simulink model "cic_filter_test9"  (Simulink 7.4)
settings: Solver=ode45  StartTime=0.0  StopTime=1000  RelTol=1e-3
libraries: xbsIndex_r4 x182, xrbsComm_r4 x1, xps_library x1, simulink x1
(part 1 of 2)
settings Model: Creator=chenhong  LastModifiedBy=chenhong

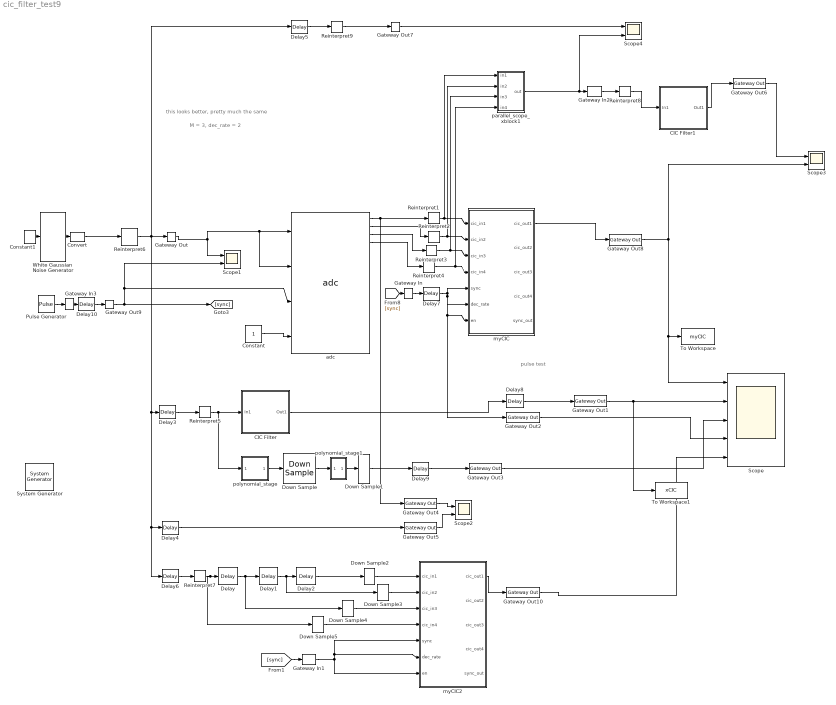
== system cic_filter_test9 ==
  note: pulse test
  note: this looks better, pretty much the same
  note: M = 3, dec_rate = 2
  " System Generator" : xbsIndex_r4/ System Generator  Tag=genX  SystemSampleTime=-1  xilinxfamily=Virtex6  part=xc6vsx315t  speed=-3  package=ff1156  synthesis_tool=XST  clock_wrapper=Clock Enables  directory=./netlist  testbench=off  simulink_period=1  sysclk_period=10  dcm_input_clock_period=10  incr_netlist=off  trim_vbits=Everywhere in SubSystem  dbl_ovrd=According to Block Masks  core_generation=According to Block Masks  run_coregen=off  deprecated_control=off  eval_field=0  block_type=sysgen
      settings: block_version=11.4
  CIC Filter : Subsystem  mask(CIC Filter){input_bitwidth=8, input_binpt=3, filter_type=Decimator, rate_change=4, stages=3, m=1, pipeline=on}
      mask prompts: input_bitwidth "Input Bit Width"; input_binpt "Input Binary Point"; filter_type "Filter Type"; rate_change "Sample Rate Change"; stages "Number of Stages"; m "Differential Delay"; pipeline "Pipeline Differentiators"
      mask help: Cascaded Integrated Comb (CIC) Filter
      mask init:
      | % CIC Single Channel v1.0
      | % Set Block Logo
      | sav_gcb=gcb;
      | [bg,fg] = xlcmap('XBlock',0);
      | iPos = get_param(sav_gcb,'Position');
      | iWidth=iPos(3)-iPos(1); iHeight=iPos(4)-iPos(2);
      | iCx=iWidth/2;
      | iCy=iHeight/2;
      | [logoX, logoY] = xlogo(iPos);
      | 
      | % Determine previous filter type and number of stages
      | prev_stages_list = find_system(sav_gcb, 'lookUnderMasks', 'all', 'FollowLinks', 'on', 'Regexp', 'on', 'Name', '^Integrator*'); %this is a cell array
      | prev_stages = length(prev_stages_list);
      | 
      | prev_filter_list = find_system(sav_gcb, 'lookUnderMasks', 'all', 'FollowLinks', 'on', 'Regexp', 'on', 'Name', '^Up Sample*'); %this is a cell array
      | if (isempty(prev_filter_list))
      |     prev_filter_list = find_system(sav_gcb, 'lookUnderMasks', 'all', 'FollowLinks', 'on', 'Regexp', 'on', 'Name', '^Down Sample*'); %this is a cell array
      |     if (isempty(prev_filter_list))
      |         errordlg('Previous Filter Type could not be determined')
      |     else
      |         prev_filter_type = 2;
      |     end
      | else
      |     prev_filter_type = 1;
      | end
      |   
      |   
      | % Print label on the block
      | if(filter_type == 2)
      |    cic_str = sprintf('%d-Stage\n CIC\n%d:1 Decimator',stages, rate_change);
      | else
      |    cic_str = sprintf('%d-Stage\n CIC\n1:%d Interpolator',stages, rate_change);	
      | end
      | 
      | % Make sure the entered values for stages and channels are positive integers
      | nstages = round(sum(abs(stages)));
      | 
      | % issue an error if the number of stages entered is zero
      | if (nstages == 0)
      | 	nstages = prev_stages;
      | 	errordlg('Number of Stages must be more than zero')
      | end
      | 
      | if (nstages == prev_stages) & (filter_type == prev_filter_type)
      |     return
      | end
      | 
      | if(filter_type == 2) % Decimator
      |    if (prev_filter_type == 1) % was interpolator so turn to decimator
      |        for i= 2:prev_stages,
      | 	      delete_line(sav_gcb, ['Integrator' int2str(i-1) '/' int2str(1)], ['Integrator' int2str(i) '/' int2str(1)]);
      | 	      delete_line(sav_gcb, ['Differentiator' int2str(i-1) '/' int2str(1)], ['Differentiator' int2str(i) '/' int2str(1)]);
      |        end
      | 
      |        % disconnect the last blocks in the two sections
      |        delete_line(sav_gcb, ['Differentiator' int2str(prev_stages) '/' int2str(1)], ['Up Sample/1']);
      |        delete_line(sav_gcb, ['Integrator' int2str(prev_stages) '/' int2str(1)], 'Out1/1');
      | 	
      | 	   % delete the line from the Up sampler to the Integrator
      | 	   delete_line(sav_gcb, 'Up Sample/1', 'Integrator1/1'); 
      | 	   delete_line(sav_gcb, 'In1/1', 'Differentiator1/1'); 
      | 	   
      | 	   % Delete the Up Sampler and then replace with an Down Sampler
      | 	   pup = get_param([sav_gcb '/Up Sample'], 'position');
      | 	   delete_block([sav_gcb '/Up Sample']);
      | 	   load_system('xbsIndex_r4');
      | 	   add_block('xbsIndex_r4/Down Sample', [sav_gcb '/Down Sample'], 'sample_ratio', 'rate_change','sample_phase', 'First Value of Frame', 'position', [pup(1), pup(2), pup(3),pup(4)]);
      | 	   
      | 	   % Switch the Integrators and Decimators around
      | 	   for i=1:prev_stages,
      | 		   tempi = get_param([sav_gcb '/Integrator' int2str(i)], 'position');
      | 	       tempd = get_param([sav_gcb '/Differentiator' int2str(i)], 'position');
      | 		   set_param([sav_gcb '/Differentiator' int2str(i)], 'position', [tempi(1), tempi(2), tempi(3), tempi(4)], 'output_bitwidth', 'ceil(stages*log2(rate_change*m) + input_bitwidth)');
      | 		   set_param([sav_gcb '/Integrator' int2str(i)], 'position', [tempd(1), tempd(2), tempd(3), tempd(4)]);
      | 	   end
      | 	   	   	
      | 	   % add back in the lines
      |        add_line(sav_gcb, 'In1/1', 'Integrator1/1', 'autorouting', 'on');
      | 	   add_line(sav_gcb, ['Integrator' int2str(prev_stages) '/1'], 'Down Sample/1', 'autorouting', 'on');
      | 	   add_line(sav_gcb, 'Down Sample/1', 'Differentiator1/1', 'autorouting', 'on');
      | 	   add_line(sav_gcb, ['Differentiator' int2str(prev_stages) '/1'], 'Out1/1', 'autorouting', 'on');
      | 	   for i= 2:prev_stages,
      |           add_line(sav_gcb, ['Integrator' int2str(i-1) '/1'], ['Integrator' int2str(i) '/' int2str(1)], 'autorouting', 'on');
      |           add_line(sav_gcb, ['Differentiator' int2str(i-1) '/1'], ['Differentiator' int2str(i) '/' int2str(1)], 'autorouting', 'on');
      | 	   end
      | 		
      |        %Set the Output bit widths of Differentiator and Integrator stages
      |        set_param([sav_gcb '/Differentiator1'], 'output_bitwidth', 'ceil(stages*log2(rate_change*m) + input_bitwidth)');
      | 	   	   %Set the Output bit width of Integrator stages
      | 	   %Calculate the Interpolator Integrator Output Bit Growth
      |        for i= 1:prev_stages,
      | 			 j = nstages+i;
      | 	         set_param([sav_gcb '/Integrator' int2str(i)], 'output_bitwidth', 'ceil(stages*log2(rate_change*m) + input_bitwidth)');
      |              set_param([sav_gcb '/Differentiator' int2str(i)], 'output_bitwidth', 'ceil(stages*log2(rate_change*m) + input_bitwidth)');
      | 	   end
      | 	   
      |    end
      |    
      |    if (nstages ~= prev_stages)
      |     
      |        % disconnect all the wires from all the blocks
      |        for i= 2:prev_stages,
      | 	      delete_line(sav_gcb, ['Integrator' int2str(i-1) '/' int2str(1)], ['Integrator' int2str(i) '/' int2str(1)]);
      | 	      delete_line(sav_gcb, ['Differentiator' int2str(i-1) '/' int2str(1)], ['Differentiator' int2str(i) '/' int2str(1)]);
      |        end
      | 
      |        % disconnect the last blocks in the two sections
      |        delete_line(sav_gcb, ['Integrator' int2str(prev_stages) '/' int2str(1)], ['Down Sample/1']);
      |        delete_line(sav_gcb, ['Differentiator' int2str(prev_stages) '/' int2str(1)], 'Out1/1');
      | 	
      | 	   % delete the line from the down sampler to the differentiator
      | 	   delete_line(sav_gcb, 'Down Sample/1', 'Differentiator1/1');
      | 	
      | 	   % Remove all the blocks except the first one (as we always will have one)
      |        for i=2:prev_stages,
      | 		  delete_block([sav_gcb '/Differentiator' int2str(i)]);
      | 	      delete_block([sav_gcb '/Integrator' int2str(i)]);
      |        end
      | 	   
      | 	   %Set the Output bit width of Differentiator stages
      |        set_param([sav_gcb '/Differentiator1'], 'output_bitwidth', 'ceil(stages*log2(rate_change*m) + input_bitwidth)');
      | 	   
      | 	   % collect data on the position of existing blocks
      | 	   pi = get_param([sav_gcb '/Integrator1'], 'position');
      | 	   pd = get_param([sav_gcb '/Differentiator1'], 'position');
      | 	   set_param([sav_gcb '/Differentiator1'], 'position', [pi(1)+(nstages+1)*80, pd(2), pi(3)+(nstages+1)*80, pd(4)]);
      | 	   pd = get_param([sav_gcb '/Differentiator1'], 'position');
      | 	
      | 	   % move the current blocks to accomadate for new blocks to be added 
      | 	   pds = get_param([sav_gcb '/Down Sample'], 'position');
      | 	   set_param([sav_gcb '/Down Sample'], 'position', [pi(1)+(nstages)*80, pds(2), pi(3)+(nstages)*80, pds(4)]);
      | 	   
      | 	   po = get_param([sav_gcb '/Out1'], 'position');
      | 	   set_param([sav_gcb '/Out1'], 'position', [pd(1)+(nstages+1)*80, po(2), pd(1)+(po(3)-po(1))+(nstages+1)*80, po(4)]);	
      | 	
      | 	   % add back in the line between the Down Sampler and the 1st Differentiator
      |        add_line(sav_gcb, 'Down Sample/1', ['Differentiator1/' int2str(1)], 'autorouting', 'on');
      | 
      | 	   % Only add blocks if more than one stage is required
      | 	   if (nstages ~= 1)
      | 		
      | 	       % Add in a copy of the first block to make up the required number of stages
      |            for i=2:nstages,
      |                add_block([sav_gcb '/Integrator1'], [sav_gcb '/Integrator' int2str(i)], 'position', [pi(1)+(i-1)*80, pi(2), pi(3)+(i-1)*80, pi(4)]);
      | 		       add_block([sav_gcb '/Differentiator1'], [sav_gcb '/Differentiator' int2str(i)], 'position', [pd(1)+(i-1)*80, pd(2), pd(3)+(i-1)*80, pd(4)]);
      | 	       end
      | 		
      | 	       % Connect up the wires to each block use autorouting
      |            for i= 2:nstages,
      |  		       add_line(sav_gcb, ['Integrator' int2str(i-1) '/' int2str(1)], ['Integrator' int2str(i) '/' int2str(1)], 'autorouting', 'on');
      | 	           add_line(sav_gcb, ['Differentiator' int2str(i-1) '/' int2str(1)], ['Differentiator' int2str(i) '/' int2str(1)], 'autorouting', 'on');
      |            end
      | 	    end
      | 	       % Connect the last blocks in the two sections
      |            add_line(sav_gcb, ['Integrator' int2str(nstages) '/' int2str(1)], ['Down Sample/1'], 'autorouting', 'on');
      |            add_line(sav_gcb, ['Differentiator' int2str(nstages) '/' int2str(1)], ['Out1/1'], 'autorouting', 'on');
      |    end
      | 
      | else % Interpolator
      |    
      | 	
      | 	if (prev_filter_type == 2) % was decimator so turn to interpolator
      | 	
      | 	  % disconnect all the wires from all the blocks
      |        for i= 2:prev_stages,
      | 	      delete_line(sav_gcb, ['Integrator' int2str(i-1) '/' int2str(1)], ['Integrator' int2str(i) '/' int2str(1)]);
      | 	      delete_line(sav_gcb, ['Differentiator' int2str(i-1) '/' int2str(1)], ['Differentiator' int2str(i) '/' int2str(1)]);
      |        end
      | 
      |        % disconnect the last blocks in the two sections
      |        delete_line(sav_gcb, ['Integrator' int2str(prev_stages) '/' int2str(1)], ['Down Sample/1']);
      |        delete_line(sav_gcb, ['Differentiator' int2str(prev_stages) '/' int2str(1)], 'Out1/1');
      | 	
      | 	   % delete the line from the down sampler to the Differentiator
      | 	   delete_line(sav_gcb, 'Down Sample/1', 'Differentiator1/1'); 
      | 	   delete_line(sav_gcb, 'In1/1', 'Integrator1/1'); 
      | 	   
      | 	   % Delete the Down Sampler and then replace with a Up Sampler
      | 	   pdwn = get_param([sav_gcb '/Down Sample'], 'position');
      | 	   delete_block([sav_gcb '/Down Sample']);
      | 	   load_system('xbsIndex_r4');
      | 	   add_block('xbsIndex_r4/Up Sample', [sav_gcb '/Up Sample'], 'sample_ratio', 'rate_change', 'position', [pdwn(1), pdwn(2), pdwn(3), pdwn(4)]);
      | 	   
      | 	   % Switch the Integrators and Decimators around
      | 	   for i=1:prev_stages,
      | 		   tempi = get_param([sav_gcb '/Integrator' int2str(i)], 'position');
      | 	       tempd = get_param([sav_gcb '/Differentiator' int2str(i)], 'position');
      | 		   set_param([sav_gcb '/Differentiator' int2str(i)], 'position', [tempi(1), tempi(2), tempi(3), tempi(4)], 'output_bitwidth', [int2str(i) '+ input_bitwidth']);
      | 		   set_param([sav_gcb '/Integrator' int2str(i)], 'position', [tempd(1), tempd(2), tempd(3), tempd(4)]);
      | 	   end
      | 	   	   	
      | 	   % add back in the lines
      |        add_line(sav_gcb, 'In1/1', 'Differentiator1/1', 'autorouting', 'on');
      | 	   add_line(sav_gcb, ['Differentiator' int2str(prev_stages) '/1'], 'Up Sample/1', 'autorouting', 'on');
      | 	   add_line(sav_gcb, 'Up Sample/1', 'Integrator1/1', 'autorouting', 'on');
      | 	   add_line(sav_gcb, ['Integrator' int2str(prev_stages) '/1'], 'Out1/1', 'autorouting', 'on');
      | 	   for i= 2:prev_stages,
      |           add_line(sav_gcb, ['Integrator' int2str(i-1) '/1'], ['Integrator' int2str(i) '/1'], 'autorouting', 'on');
      |           add_line(sav_gcb, ['Differentiator' int2str(i-1) '/1'], ['Differentiator' int2str(i) '/1'], 'autorouting', 'on');
      | 	   end
      | 	   
      | 	   %Set the Output bit width of Integrator stages
      | 	   %Calculate the Interpolator Integrator Output Bit Growth
      |        for i= 1:prev_stages,
      | 			 j = nstages+i;
      | 	         set_param([sav_gcb '/Integrator' int2str(i)], 'output_bitwidth', ['ceil(log2(2^(2*stages-' int2str(j) ')*(rate_change*m)^(' int2str(j) '-stages)) + input_bitwidth)']);
      | 	   end
      | 		
      |    end
      |    
      | 	
      | 	if (nstages ~= prev_stages)
      |     
      |        % disconnect all the wires from all the blocks
      |        for i= 2:prev_stages,
      | 	      delete_line(sav_gcb, ['Integrator' int2str(i-1) '/' int2str(1)], ['Integrator' int2str(i) '/' int2str(1)]);
      | 	      delete_line(sav_gcb, ['Differentiator' int2str(i-1) '/' int2str(1)], ['Differentiator' int2str(i) '/' int2str(1)]);
      |        end
      | 
      |        % disconnect the last blocks in the two sections
      |        delete_line(sav_gcb, ['Differentiator' int2str(prev_stages) '/' int2str(1)], ['Up Sample/1']);
      |        delete_line(sav_gcb, ['Integrator' int2str(prev_stages) '/' int2str(1)], 'Out1/1');
      |        
      | 	
      | 	   % delete the line from the Up sampler to the Integrator1 for movement later
      | 	   delete_line(sav_gcb, 'Up Sample/1', 'Integrator1/1'); 
      | 	
      | 	   % Remove all the blocks except the first one (as we always will have one)
      |        for i=2:prev_stages,
      | 		  delete_block([sav_gcb '/Differentiator' int2str(i)]);
      | 	      delete_block([sav_gcb '/Integrator' int2str(i)]);
      |        end
      | 	
      | 	   %Set the Output bit width of first Differentiator stage (other are set as copies of this block)
      |        set_param([sav_gcb '/Differentiator1'], 'output_bitwidth', '1 + input_bitwidth');
      | 	   
      | 	   % collect data on the position of existing blocks
      | 	   pi = get_param([sav_gcb '/Integrator1'], 'position');
      | 	   pd = get_param([sav_gcb '/Differentiator1'], 'position');
      | 	   set_param([sav_gcb '/Integrator1'], 'position', [pd(1)+(nstages+1)*80, pi(2), pd(3)+(nstages+1)*80, pi(4)]);
      | 	   pi = get_param([sav_gcb '/Integrator1'], 'position');
      | 	
      | 	   % move the current blocks to accomadate for new blocks to be added 
      | 	   pus = get_param([sav_gcb '/Up Sample'], 'position');
      | 	   set_param([sav_gcb '/Up Sample'], 'position', [pd(1)+(nstages)*80, pus(2), pd(3)+(nstages)*80, pus(4)]);
      | 	
      | 	   po = get_param([sav_gcb '/Out1'], 'position');
      |        set_param([sav_gcb '/Out1'], 'position', [pi(1)+(nstages+1)*80, po(2), pi(1)+(po(3)-po(1))+(nstages+1)*80, po(4)]);	
      |       
      | 	
      | 	   % add back in the line between the Up Sampler and the 1st Integrator1
      | 	   add_line(sav_gcb, 'Up Sample/1', 'Integrator1/1', 'autorouting', 'on');
      | 	   
      | 	   % Only add blocks if more than one stage is required
      | 	   if (nstages ~= 1)
      | 		
      | 	       % Add in a copy of the first block to make up the required number of stages
      |            for i=2:nstages,
      |                add_block([sav_gcb '/Integrator1'], [sav_gcb '/Integrator' int2str(i)], 'position', [pi(1)+(i-1)*80, pi(2), pi(3)+(i-1)*80, pi(4)]);
      | 		       add_block([sav_gcb '/Differentiator1'], [sav_gcb '/Differentiator' int2str(i)], 'position', [pd(1)+(i-1)*80, pd(2), pd(3)+(i-1)*80, pd(4)], 'output_bitwidth', [int2str(i) '+ input_bitwidth']);
      | 	       end
      | 		
      | 	       % Connect up the wires to each block use autorouting
      |            for i= 2:nstages,
      |  		       add_line(sav_gcb, ['Integrator' int2str(i-1) '/' int2str(1)], ['Integrator' int2str(i) '/' int2str(1)], 'autorouting', 'on');
      | 	           add_line(sav_gcb, ['Differentiator' int2str(i-1) '/' int2str(1)], ['Differentiator' int2str(i) '/' int2str(1)], 'autorouting', 'on');
      |            end
      | 	    end
      | 	       % Connect the last blocks in the two sections
      |            add_line(sav_gcb, ['Differentiator' int2str(nstages) '/1'], ['Up Sample/1'], 'autorouting', 'on');
      |            add_line(sav_gcb, ['Integrator' int2str(nstages) '/1'], ['Out1/1'], 'autorouting', 'on');
      | 		   
      | 	     %Set the Output bit width of Integrator stages
      | 	     %Calculate the Interpolator Integrator Output Bit Growth
      |           for i= 1:nstages,
      | 			 j = nstages+i;
      | 	         set_param([sav_gcb '/Integrator' int2str(i)], 'output_bitwidth', ['ceil(log2(2^(2*stages-' int2str(j) ')*(rate_change*m)^(' int2str(j) '-stages)) + input_bitwidth)']);
      | 	      end
      |    end
      | 	  
      | end
      | 
      | 
      | % Set the pipelining to ON or OFF on the differentiators
      | if (pipeline == 0)
      | 	for i= 1:nstages
      | 		set_param([sav_gcb '/Differentiator' int2str(i), '/AddSub'], 'latency', '0')
      | 	end
      | else
      | 	for i= 1:nstages
      | 		set_param([sav_gcb '/Differentiator' int2str(i), '/AddSub'], 'latency' ,'1')
      | 	end
      | end
      settings: CopyFcn=set_param(gcb, 'MaskSelfModifiable', 'on', 'LinkStatus', 'none');
      mask Help: eval('');xlDoc('-book','sysgen','-topic','CIC_Filter');
      mask StyleString: edit,edit,popup(Interpolator|Decimator),edit,edit,popup(1|2|3|4),checkbox
      mask Display:
      | patch([0 iWidth iWidth 0],[0 0 iHeight iHeight] , bg);
      | patch(logoX,logoY , fg);
      | plot([0 0 iWidth iWidth 0], [0 iHeight iHeight 0 0]);
      | disp(cic_str)
  CIC Filter1 : Subsystem  mask(CIC Filter){input_bitwidth=8, input_binpt=3, filter_type=Decimator, rate_change=2, stages=3, m=1, pipeline=on}
      mask prompts: input_bitwidth "Input Bit Width"; input_binpt "Input Binary Point"; filter_type "Filter Type"; rate_change "Sample Rate Change"; stages "Number of Stages"; m "Differential Delay"; pipeline "Pipeline Differentiators"
      mask help: Cascaded Integrated Comb (CIC) Filter
      mask init: same as cic_filter_test9/CIC Filter
      settings: CopyFcn=set_param(gcb, 'MaskSelfModifiable', 'on', 'LinkStatus', 'none');
      mask Help: eval('');xlDoc('-book','sysgen','-topic','CIC_Filter');
      mask StyleString: edit,edit,popup(Interpolator|Decimator),edit,edit,popup(1|2|3|4),checkbox
      mask Display:
      | patch([0 iWidth iWidth 0],[0 0 iHeight iHeight] , bg);
      | patch(logoX,logoY , fg);
      | plot([0 0 iWidth iWidth 0], [0 iHeight iHeight 0 0]);
      | disp(cic_str)
  Constant : Constant  OutDataType=fixdt(1, 16)  OutScaling=2^0
  Constant1 : xbsIndex_r4/Constant  arith_type=Boolean  const=0  n_bits=16  bin_pt=14  explicit_period=on  period=1  equ=P=C  opselect=C  inp2=PCIN>>17  opr=+  inp1=P  carry=CIN  dbl_ovrd=off  block_type=constant
      settings: block_version=11.4
  Convert : xbsIndex_r4/Convert  arith_type="Signed  (2's comp)"  n_bits=8  bin_pt=7  quantization=Truncate  overflow=Wrap  latency=0  dbl_ovrd=off  pipeline=off  block_type=convert
      settings: block_version=11.4
  Delay : xbsIndex_r4/Delay  en=off  latency=1  dbl_ovrd=off  reg_retiming=off  block_type=delay
      settings: block_version=11.4
  Delay1 : xbsIndex_r4/Delay  en=off  latency=1  dbl_ovrd=off  reg_retiming=off  block_type=delay
      settings: block_version=11.4
  Delay10 : xbsIndex_r4/Delay  en=off  latency=50  dbl_ovrd=off  reg_retiming=off  block_type=delay
      settings: block_version=11.4
  Delay2 : xbsIndex_r4/Delay  en=off  latency=1  dbl_ovrd=off  reg_retiming=off  block_type=delay
      settings: block_version=11.4
  Delay{3..6} (4 alike) : xbsIndex_r4/Delay  en=off  latency=8  dbl_ovrd=off  reg_retiming=off  block_type=delay
      settings: block_version=11.4
  Delay7 : xbsIndex_r4/Delay  en=off  latency=50  dbl_ovrd=off  reg_retiming=off  block_type=delay
      settings: block_version=11.4
  Delay8 : xbsIndex_r4/Delay  en=off  latency=2  dbl_ovrd=off  reg_retiming=off  block_type=delay
      settings: block_version=11.4
  Delay9 : xbsIndex_r4/Delay  en=off  latency=5  dbl_ovrd=off  reg_retiming=off  block_type=delay
      settings: block_version=11.4
  Down Sample : xbsIndex_r4/Down Sample  sample_ratio=2  sample_phase="Last Value of Frame  (most efficient)"  en=off  latency=1  dbl_ovrd=off  block_type=dsamp
      settings: block_version=11.4
  Down Sample1 : xbsIndex_r4/Down Sample  sample_ratio=2  sample_phase="Last Value of Frame  (most efficient)"  en=off  latency=1  dbl_ovrd=off  block_type=dsamp
      settings: block_version=11.4
  Down Sample{2..5} (4 alike) : xbsIndex_r4/Down Sample  sample_ratio=4  sample_phase="Last Value of Frame  (most efficient)"  en=off  latency=1  dbl_ovrd=off  block_type=dsamp
      settings: block_version=11.4
  Gateway In : xbsIndex_r4/Gateway In  arith_type=Boolean  n_bits=16  bin_pt=14  quantization="Round  (unbiased: +/- Inf)"  overflow=Saturate  period=1  dbl_ovrd=off  timing_constraint=None  locs_specified=off  LOCs={}  hdl_port=on  block_type=gatewayin
      settings: infoedit="Gateway in block.  Converts inputs of type Simulink integer, double and fixed point to  Xilinx fixed point type.<br><br>Hardware notes:  In hardware these blocks become top level input ports."  block_version=11.4
  Gateway In1 : xbsIndex_r4/Gateway In  arith_type=Boolean  n_bits=16  bin_pt=14  quantization="Round  (unbiased: +/- Inf)"  overflow=Saturate  period=1  dbl_ovrd=off  timing_constraint=None  locs_specified=off  LOCs={}  hdl_port=on  block_type=gatewayin
      settings: infoedit="Gateway in block.  Converts inputs of type Simulink integer, double and fixed point to  Xilinx fixed point type.<br><br>Hardware notes:  In hardware these blocks become top level input ports."  block_version=11.4
  Gateway In2 : xbsIndex_r4/Gateway In  arith_type="Signed  (2's comp)"  n_bits=8  bin_pt=7  quantization="Round  (unbiased: +/- Inf)"  overflow=Saturate  period=1  dbl_ovrd=off  timing_constraint=None  locs_specified=off  LOCs={}  hdl_port=on  block_type=gatewayin
      settings: infoedit="Gateway in block.  Converts inputs of type Simulink integer, double and fixed point to  Xilinx fixed point type.<br><br>Hardware notes:  In hardware these blocks become top level input ports."  block_version=11.4
  Gateway In3 : xbsIndex_r4/Gateway In  arith_type=Boolean  n_bits=16  bin_pt=14  quantization="Round  (unbiased: +/- Inf)"  overflow=Saturate  period=1  dbl_ovrd=off  timing_constraint=None  locs_specified=off  LOCs={}  hdl_port=on  block_type=gatewayin
      settings: infoedit="Gateway in block.  Converts inputs of type Simulink integer, double and fixed point to  Xilinx fixed point type.<br><br>Hardware notes:  In hardware these blocks become top level input ports."  block_version=11.4
  Gateway Out{,1..7,9} (9 alike) : xbsIndex_r4/Gateway Out  hdl_port=on  timing_constraint=None  locs_specified=off  LOCs={}  block_type=gatewayout
      settings: infoedit="Gateway out block.  Converts Xilinx fixed point inputs into ouputs of type Simulink integer, double, or fixed point.<br><br>Hardware notes:  In hardware these blocks become top level output ports or are discarded, depending on how they are configured."  block_version=11.4
  Gateway Out10 : xbsIndex_r4/Gateway Out  hdl_port=off  timing_constraint=None  locs_specified=off  LOCs={}  block_type=gatewayout
      settings: infoedit="Gateway out block.  Converts Xilinx fixed point inputs into ouputs of type Simulink integer, double, or fixed point.<br><br>Hardware notes:  In hardware these blocks become top level output ports or are discarded, depending on how they are configured."  block_version=11.4
  Gateway Out8 : xbsIndex_r4/Gateway Out  hdl_port=off  timing_constraint=None  locs_specified=off  LOCs={}  block_type=gatewayout
      settings: infoedit="Gateway out block.  Converts Xilinx fixed point inputs into ouputs of type Simulink integer, double, or fixed point.<br><br>Hardware notes:  In hardware these blocks become top level output ports or are discarded, depending on how they are configured."  block_version=11.4
  Pulse Generator : DiscretePulseGenerator  Amplitude=1  Period=2  PulseWidth=1  PhaseDelay=0  SampleTime=1
  Reinterpret{1..5,7..9} (8 alike) : xbsIndex_r4/Reinterpret  force_arith_type=on  arith_type="Signed  (2's comp)"  force_bin_pt=on  bin_pt=3  block_type=reinterpret
      settings: infoedit="Changes signal type without altering the binary representation.   You can changed the signal between signed and unsigned, and relocate the binary point.<br><br>Hardware notes: In hardware this block costs nothing.<br><br>Example:  Suppose the input is 6 bits wide, signed, with 2 fractional bits, and the output is forced to unsigned with 0 fractional bits.  Then an input of -2.0 (1110.00 in binary 2's complement) becomes an output of 56 (111000 in binary)."
  Reinterpret6 : xbsIndex_r4/Reinterpret  force_arith_type=on  arith_type="Signed  (2's comp)"  force_bin_pt=on  bin_pt=7  block_type=reinterpret
      settings: infoedit="Changes signal type without altering the binary representation.   You can changed the signal between signed and unsigned, and relocate the binary point.<br><br>Hardware notes: In hardware this block costs nothing.<br><br>Example:  Suppose the input is 6 bits wide, signed, with 2 fractional bits, and the output is forced to unsigned with 0 fractional bits.  Then an input of -2.0 (1110.00 in binary 2's complement) becomes an output of 56 (111000 in binary)."
  Scope : Scope  NumInputPorts=5
      settings: YMin=-5~-5~-5~-5~-5  YMax=5~5~5~5~5
  Scope{1..4} (4 alike) : Scope  NumInputPorts=2
      Scope1 settings: TimeRange=1000  YMin=0~0  YMax=2~1
      Scope2 settings: TimeRange=1000  YMin=0~-5  YMax=2~5  SaveName=ScopeData2
      Scope3 settings: TimeRange=1000  YMin=0~0  YMax=2~1  SaveName=ScopeData3
      Scope4 settings: TimeRange=1000  YMin=0~0  YMax=2~1  SaveName=ScopeData4
  To Workspace : ToWorkspace  VariableName=myCIC  SampleTime=-1  SaveFormat=Structure
  To Workspace1 : ToWorkspace  VariableName=xCIC  SampleTime=-1  SaveFormat=Structure
  White Gaussian  Noise Generator : xrbsComm_r4/White Gaussian  Noise Generator  SystemSampleTime=-1  seed=512
  adc : xps_library/adc  Tag=xps:adc  SystemSampleTime=-1  adc_brd=adc0  adc_clk_rate=800  adc_interleave=off  sample_period=4
  myCIC : Subsystem
  myCIC2 : Subsystem
  parallel_scope_xblock1 : Subsystem  mask(dsp_scope){n_inputs=4, sample_period=4}
      mask prompts: n_inputs "Number of inputs"; sample_period "Sample Period"
      mask help:
      | This block provides a convenient interface to plotting waveforms
      | of blocks with serial data output in parallel.  The core example
      | is of the ADC, which outputs 8 samples / clock.  This scope (simulation only)
      | samples sufficently fast (based on the number of parallel inputs)
      | to serialize the output for view in a standard simulink scope.
      |
      | The input must be concatenated parallel data streams, and
      | each data binary point must be 0.  The easiest way to do this is
      | to push  all the inputs through a "cram" block from the
      | GAVRT blockset.
      | easy
      mask init:
      | config.source = str2func('parallel_scope_init_xblock');
      | config.toplevel = gcb;
      | xBlock(config, ...
      |     {'n_inputs', n_inputs, ...
      |     'sample_period', sample_period});
  polynomial_stage : Subsystem
  polynomial_stage1 : Subsystem
  wires:
  Constant/1 -> adc/4
  Pulse Generator/1 -> Gateway In3/1
  Gateway Out/1 -> Scope1/1, adc/1, adc/2
  Reinterpret6/1 -> Gateway Out/1, Delay4/1, Delay6/1, Delay3/1, Delay5/1
  adc/1 -> Reinterpret1/1, Gateway Out4/1
  adc/2 -> Reinterpret2/1
  adc/3 -> Reinterpret3/1
  adc/4 -> Reinterpret4/1
  [sync] -> Gateway In/1
  myCIC/1(cic_out1) -> Gateway Out8/1
  CIC Filter/1(Out1) -> Delay8/1
  Gateway Out1/1 -> Scope/2, To Workspace1/1
  Gateway In/1 -> Delay7/1
  Reinterpret1/1 -> myCIC/1(cic_in1), parallel_scope_xblock1/1(in1)
  Reinterpret2/1 -> myCIC/2(cic_in2), parallel_scope_xblock1/2(in2)
  Reinterpret3/1 -> myCIC/3(cic_in3), parallel_scope_xblock1/3(in3)
  Reinterpret4/1 -> myCIC/4(cic_in4), parallel_scope_xblock1/4(in4)
  Reinterpret5/1 -> CIC Filter/1(In1), polynomial_stage/1(inport)
  polynomial_stage/1(outport) -> Down Sample/1
  Gateway Out3/1 -> Scope/3
  Gateway Out2/1 -> Scope/4
  Gateway Out4/1 -> Scope2/1
  Gateway Out5/1 -> Scope2/2
  White Gaussian  Noise Generator/1 -> Convert/1
  Constant1/1 -> White Gaussian  Noise Generator/1
  Delay/1 -> Delay1/1, Down Sample4/1
  Delay1/1 -> Delay2/1, Down Sample3/1
  Delay2/1 -> Down Sample2/1
  [sync] -> Gateway In1/1
  Gateway In1/1 -> myCIC2/6(dec_rate), myCIC2/5(sync), myCIC2/7(en)
  myCIC2/1(cic_out1) -> Gateway Out10/1
  Reinterpret7/1 -> Delay/1, Down Sample5/1
  Convert/1 -> Reinterpret6/1
  parallel_scope_xblock1/1(out) -> Gateway In2/1, Scope4/2
  Reinterpret8/1 -> CIC Filter1/1(In1)
  CIC Filter1/1(Out1) -> Gateway Out6/1
  Gateway Out6/1 -> Scope3/1
  Gateway In2/1 -> Reinterpret8/1
  Delay3/1 -> Reinterpret5/1
  Delay4/1 -> Gateway Out5/1
  Delay5/1 -> Reinterpret9/1
  Delay6/1 -> Reinterpret7/1
  Delay7/1 -> Gateway Out2/1, myCIC/7(en), myCIC/6(dec_rate), myCIC/5(sync)
  Gateway Out7/1 -> Scope4/1
  Reinterpret9/1 -> Gateway Out7/1
  Down Sample/1 -> polynomial_stage1/1(inport)
  Delay8/1 -> Gateway Out1/1
  Delay9/1 -> Gateway Out3/1
  polynomial_stage1/1(outport) -> Down Sample1/1
  Down Sample1/1 -> Delay9/1
  Gateway Out8/1 -> Scope/1, To Workspace/1, Scope3/2
  Delay10/1 -> Gateway Out9/1
  Gateway In3/1 -> Delay10/1
  Gateway Out9/1 -> Scope1/2, adc/3, [sync]
  Gateway Out10/1 -> Scope/5
  Down Sample3/1 -> myCIC2/2(cic_in2)
  Down Sample2/1 -> myCIC2/1(cic_in1)
  Down Sample4/1 -> myCIC2/3(cic_in3)
  Down Sample5/1 -> myCIC2/4(cic_in4)

== system cic_filter_test9/CIC Filter ==
  note: The CIC filter is constructed out of differentiators and integrators and
      | a sample rate change. This block provides a full precision result and is
      | dynamically built given the parameters entered in the dialog box. The
      | dynamic rebuilding script can switch which side the integrators and
      | differentiators are on and also change between an up and down sampler
      | depending on whether an Interpolator or decimator is selected respectively.
      | The number of stages selected control how many integrators and
      | differentiators are used.
  note: The Interpoiation by 48, 4 stage CIC filter occupies 116 slices.
      | The maximum clock frequency is approximately
      | 308.55 MHz in a Xilinx xc2vp2-7 part (Device speed data version:
      | PRODUCTION 1.121 2005-11-04, ISE 8.1.01i I.25 software, VHDL
      | synthesized with XST).
  In1 : Inport  OutDataType=sfix(16)  OutScaling=2^0
  Differentiator1 : Subsystem  mask(Differentiator Stage){m=m, output_bitwidth=ceil(stages*log2(rate_change*m) + input_bitwidth), output_binpt=input_binpt}
      mask prompts: m "Differential Delay"; output_bitwidth "Output Bit Width"; output_binpt "Output Binary Point"
      mask help: Multi-Channel Differentiator
      mask init:
      | set_param(gcb, 'LinkStatus', 'none');
  Differentiator2 : Subsystem  mask(Differentiator Stage){m=m, output_bitwidth=ceil(stages*log2(rate_change*m) + input_bitwidth), output_binpt=input_binpt}
      mask prompts: m "Differential Delay"; output_bitwidth "Output Bit Width"; output_binpt "Output Binary Point"
      mask help: Multi-Channel Differentiator
      mask init:
      | set_param(gcb, 'LinkStatus', 'none');
  Differentiator3 : Subsystem  mask(Differentiator Stage){m=m, output_bitwidth=ceil(stages*log2(rate_change*m) + input_bitwidth), output_binpt=input_binpt}
      mask prompts: m "Differential Delay"; output_bitwidth "Output Bit Width"; output_binpt "Output Binary Point"
      mask help: Multi-Channel Differentiator
      mask init:
      | set_param(gcb, 'LinkStatus', 'none');
  Down Sample : xbsIndex_r4/Down Sample  sample_ratio=rate_change  sample_phase=First Value of Frame  en=off  latency=1  dbl_ovrd=off  block_type=dsamp
      settings: block_version=9.2.00
  Integrator1 : Subsystem  mask(Integrator Stage){output_bitwidth=ceil(stages*log2(rate_change*m) + input_bitwidth)}
      mask prompts: output_bitwidth "Output Bit Width"
      mask help: Multi Channel Integrator
      mask init:
      | set_param(gcb, 'LinkStatus', 'none');
      settings: CopyFcn=set_param(gcb, 'LinkStatus', 'none');
  Integrator2 : Subsystem  mask(Integrator Stage){output_bitwidth=ceil(stages*log2(rate_change*m) + input_bitwidth)}
      mask prompts: output_bitwidth "Output Bit Width"
      mask help: Multi Channel Integrator
      mask init:
      | set_param(gcb, 'LinkStatus', 'none');
      settings: CopyFcn=set_param(gcb, 'LinkStatus', 'none');
  Integrator3 : Subsystem  mask(Integrator Stage){output_bitwidth=ceil(stages*log2(rate_change*m) + input_bitwidth)}
      mask prompts: output_bitwidth "Output Bit Width"
      mask help: Multi Channel Integrator
      mask init:
      | set_param(gcb, 'LinkStatus', 'none');
      settings: CopyFcn=set_param(gcb, 'LinkStatus', 'none');
  Out1 : Outport  OutDataType=sfix(16)  OutScaling=2^0
  wires:
  In1/1 -> Integrator1/1(In1)
  Down Sample/1 -> Differentiator1/1(In1)
  Integrator1/1(Out1) -> Integrator2/1(In1)
  Differentiator1/1(Out1) -> Differentiator2/1(In1)
  Integrator2/1(Out1) -> Integrator3/1(In1)
  Differentiator2/1(Out1) -> Differentiator3/1(In1)
  Integrator3/1(Out1) -> Down Sample/1
  Differentiator3/1(Out1) -> Out1/1

== system cic_filter_test9/CIC Filter1 ==
  note: The CIC filter is constructed out of differentiators and integrators and
      | a sample rate change. This block provides a full precision result and is
      | dynamically built given the parameters entered in the dialog box. The
      | dynamic rebuilding script can switch which side the integrators and
      | differentiators are on and also change between an up and down sampler
      | depending on whether an Interpolator or decimator is selected respectively.
      | The number of stages selected control how many integrators and
      | differentiators are used.
  note: The Interpoiation by 48, 4 stage CIC filter occupies 116 slices.
      | The maximum clock frequency is approximately
      | 308.55 MHz in a Xilinx xc2vp2-7 part (Device speed data version:
      | PRODUCTION 1.121 2005-11-04, ISE 8.1.01i I.25 software, VHDL
      | synthesized with XST).
  In1 : Inport  OutDataType=sfix(16)  OutScaling=2^0
  Differentiator1 : Subsystem  mask(Differentiator Stage){m=m, output_bitwidth=ceil(stages*log2(rate_change*m) + input_bitwidth), output_binpt=input_binpt}
      mask prompts: m "Differential Delay"; output_bitwidth "Output Bit Width"; output_binpt "Output Binary Point"
      mask help: Multi-Channel Differentiator
      mask init:
      | set_param(gcb, 'LinkStatus', 'none');
  Differentiator2 : Subsystem  mask(Differentiator Stage){m=m, output_bitwidth=ceil(stages*log2(rate_change*m) + input_bitwidth), output_binpt=input_binpt}
      mask prompts: m "Differential Delay"; output_bitwidth "Output Bit Width"; output_binpt "Output Binary Point"
      mask help: Multi-Channel Differentiator
      mask init:
      | set_param(gcb, 'LinkStatus', 'none');
  Differentiator3 : Subsystem  mask(Differentiator Stage){m=m, output_bitwidth=ceil(stages*log2(rate_change*m) + input_bitwidth), output_binpt=input_binpt}
      mask prompts: m "Differential Delay"; output_bitwidth "Output Bit Width"; output_binpt "Output Binary Point"
      mask help: Multi-Channel Differentiator
      mask init:
      | set_param(gcb, 'LinkStatus', 'none');
  Down Sample : xbsIndex_r4/Down Sample  sample_ratio=rate_change  sample_phase=First Value of Frame  en=off  latency=1  dbl_ovrd=off  block_type=dsamp
      settings: block_version=9.2.00
  Integrator1 : Subsystem  mask(Integrator Stage){output_bitwidth=ceil(stages*log2(rate_change*m) + input_bitwidth)}
      mask prompts: output_bitwidth "Output Bit Width"
      mask help: Multi Channel Integrator
      mask init:
      | set_param(gcb, 'LinkStatus', 'none');
      settings: CopyFcn=set_param(gcb, 'LinkStatus', 'none');
  Integrator2 : Subsystem  mask(Integrator Stage){output_bitwidth=ceil(stages*log2(rate_change*m) + input_bitwidth)}
      mask prompts: output_bitwidth "Output Bit Width"
      mask help: Multi Channel Integrator
      mask init:
      | set_param(gcb, 'LinkStatus', 'none');
      settings: CopyFcn=set_param(gcb, 'LinkStatus', 'none');
  Integrator3 : Subsystem  mask(Integrator Stage){output_bitwidth=ceil(stages*log2(rate_change*m) + input_bitwidth)}
      mask prompts: output_bitwidth "Output Bit Width"
      mask help: Multi Channel Integrator
      mask init:
      | set_param(gcb, 'LinkStatus', 'none');
      settings: CopyFcn=set_param(gcb, 'LinkStatus', 'none');
  Out1 : Outport  OutDataType=sfix(16)  OutScaling=2^0
  wires:
  In1/1 -> Integrator1/1(In1)
  Down Sample/1 -> Differentiator1/1(In1)
  Integrator1/1(Out1) -> Integrator2/1(In1)
  Differentiator1/1(Out1) -> Differentiator2/1(In1)
  Integrator2/1(Out1) -> Integrator3/1(In1)
  Differentiator2/1(Out1) -> Differentiator3/1(In1)
  Integrator3/1(Out1) -> Down Sample/1
  Differentiator3/1(Out1) -> Out1/1

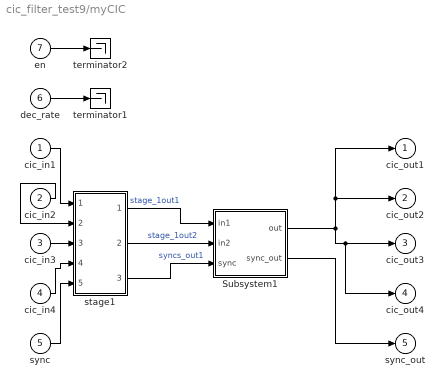
== system cic_filter_test9/myCIC ==
  cic_in1 : Inport
  cic_in2 : Inport  Port=2
  cic_in3 : Inport  Port=3
  cic_in4 : Inport  Port=4
  sync : Inport  Port=5
  dec_rate : Inport  Port=6
  en : Inport  Port=7
  Subsystem1 : Subsystem
  stage1 : Subsystem
  terminator1 : Terminator
  terminator2 : Terminator
  cic_out1 : Outport
  cic_out2 : Outport  Port=2
  cic_out3 : Outport  Port=3
  cic_out4 : Outport  Port=4
  sync_out : Outport  Port=5
  wires:
  sync/1 -> stage1/5(sync)
  cic_in3/1 -> stage1/3(inport3)
  cic_in1/1 -> stage1/1(inport1)
  en/1 -> terminator2/1
  dec_rate/1 -> terminator1/1
  cic_in2/1 -> stage1/2(inport2)
  cic_in4/1 -> stage1/4(inport4)
  stage1/1(outport2) -> Subsystem1/1(in1)  "stage_1out1"
  stage1/2(outport4) -> Subsystem1/2(in2)  "stage_1out2"
  stage1/3(sync_out) -> Subsystem1/3(sync)  "syncs_out1"
  Subsystem1/2(sync_out) -> sync_out/1
  Subsystem1/1(out) -> cic_out1/1, cic_out2/1, cic_out3/1, cic_out4/1

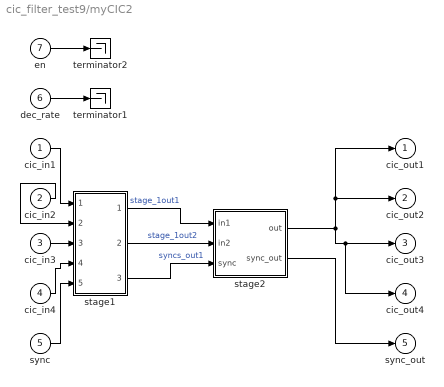
== system cic_filter_test9/myCIC2 ==
  cic_in1 : Inport
  cic_in2 : Inport  Port=2
  cic_in3 : Inport  Port=3
  cic_in4 : Inport  Port=4
  sync : Inport  Port=5
  dec_rate : Inport  Port=6
  en : Inport  Port=7
  stage1 : Subsystem
  stage2 : Subsystem
  terminator1 : Terminator
  terminator2 : Terminator
  cic_out1 : Outport
  cic_out2 : Outport  Port=2
  cic_out3 : Outport  Port=3
  cic_out4 : Outport  Port=4
  sync_out : Outport  Port=5
  wires:
  sync/1 -> stage1/5(sync)
  cic_in3/1 -> stage1/3(inport3)
  cic_in1/1 -> stage1/1(inport1)
  en/1 -> terminator2/1
  dec_rate/1 -> terminator1/1
  cic_in2/1 -> stage1/2(inport2)
  cic_in4/1 -> stage1/4(inport4)
  stage1/1(outport2) -> stage2/1(in1)  "stage_1out1"
  stage1/2(outport4) -> stage2/2(in2)  "stage_1out2"
  stage1/3(sync_out) -> stage2/3(sync)  "syncs_out1"
  stage2/2(sync_out) -> sync_out/1
  stage2/1(out) -> cic_out1/1, cic_out2/1, cic_out3/1, cic_out4/1

== system cic_filter_test9/parallel_scope_xblock1 ==
  in1 : Inport
  in2 : Inport  Port=2
  in3 : Inport  Port=3
  in4 : Inport  Port=4
  gateway_out{1..4} (4 alike) : xbsIndex_r4/Gateway Out  hdl_port=off  timing_constraint=None  locs_specified=off  LOCs={}  block_type=gatewayout
      settings: infoedit="Gateway out block.  Converts Xilinx fixed point inputs into ouputs of type Simulink integer, double, or fixed point.<br><br>Hardware notes:  In hardware these blocks become top level output ports or are discarded, depending on how they are configured."  block_version=11.4
  sel : simulink/Sources/Counter Free-Running  SystemSampleTime=-1  NumBits=2  tsamp=1
  switch : MultiPortSwitch  Inputs=4  zeroidx=on  OutDataType=fixdt(1, 16)  OutScaling=2^0
  out : Outport
  wires:
  switch/1 -> out/1
  gateway_out4/1 -> switch/5  "switcher_in4"
  gateway_out3/1 -> switch/4  "switcher_in3"
  gateway_out2/1 -> switch/3  "switcher_in2"
  gateway_out1/1 -> switch/2  "switcher_in1"
  sel/1 -> switch/1  "sel_out"
  in4/1 -> gateway_out4/1
  in3/1 -> gateway_out3/1
  in2/1 -> gateway_out2/1
  in1/1 -> gateway_out1/1

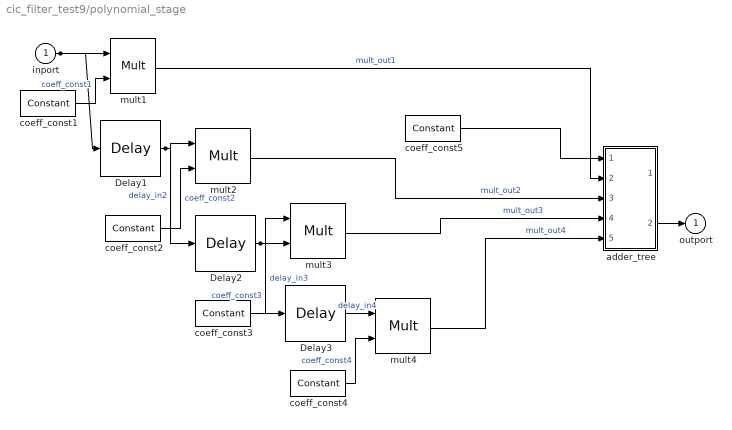
== system cic_filter_test9/polynomial_stage ==
  inport : Inport
  Delay1 : xbsIndex_r4/Delay  en=off  latency=1  dbl_ovrd=off  reg_retiming=off  block_type=delay
      settings: block_version=11.4
  Delay2 : xbsIndex_r4/Delay  en=off  latency=1  dbl_ovrd=off  reg_retiming=off  block_type=delay
      settings: block_version=11.4
  Delay3 : xbsIndex_r4/Delay  en=off  latency=1  dbl_ovrd=off  reg_retiming=off  block_type=delay
      settings: block_version=11.4
  adder_tree : Subsystem
  coeff_const1 : xbsIndex_r4/Constant  arith_type=Signed (2's comp)  const=1  n_bits=3  bin_pt=0  explicit_period=off  period=1  equ=P=C  opselect=C  inp2=PCIN>>17  opr=+  inp1=P  carry=CIN  dbl_ovrd=off  block_type=constant
      settings: block_version=11.4
  coeff_const2 : xbsIndex_r4/Constant  arith_type=Signed (2's comp)  const=3  n_bits=3  bin_pt=0  explicit_period=off  period=1  equ=P=C  opselect=C  inp2=PCIN>>17  opr=+  inp1=P  carry=CIN  dbl_ovrd=off  block_type=constant
      settings: block_version=11.4
  coeff_const3 : xbsIndex_r4/Constant  arith_type=Signed (2's comp)  const=3  n_bits=3  bin_pt=0  explicit_period=off  period=1  equ=P=C  opselect=C  inp2=PCIN>>17  opr=+  inp1=P  carry=CIN  dbl_ovrd=off  block_type=constant
      settings: block_version=11.4
  coeff_const4 : xbsIndex_r4/Constant  arith_type=Signed (2's comp)  const=1  n_bits=3  bin_pt=0  explicit_period=off  period=1  equ=P=C  opselect=C  inp2=PCIN>>17  opr=+  inp1=P  carry=CIN  dbl_ovrd=off  block_type=constant
      settings: block_version=11.4
  coeff_const5 : xbsIndex_r4/Constant  arith_type=Boolean  const=1  n_bits=6  bin_pt=0  explicit_period=on  period=1  equ=P=C  opselect=C  inp2=PCIN>>17  opr=+  inp1=P  carry=CIN  dbl_ovrd=off  block_type=constant
      settings: block_version=11.4
  mult{1..4} (4 alike) : xbsIndex_r4/Mult  precision=Full  arith_type="Signed  (2's comp)"  n_bits=9  bin_pt=0  quantization=Truncate  overflow=Wrap  en=off  latency=2  dbl_ovrd=off  use_behavioral_HDL=off  opt=Speed  use_embedded=on  optimum_pipeline=off  pipeline=on  use_rpm=on  placement_style=Triangular  block_type=mult
      settings: block_version=11.4
  outport : Outport
  wires:
  inport/1 -> Delay1/1, mult1/1
  Delay1/1 -> mult2/1, Delay2/1  "delay_in2"
  Delay2/1 -> Delay3/1, mult3/1  "delay_in3"
  Delay3/1 -> mult4/1  "delay_in4"
  coeff_const3/1 -> mult3/2  "coeff_const3"
  coeff_const1/1 -> mult1/2  "coeff_const1"
  coeff_const2/1 -> mult2/2  "coeff_const2"
  coeff_const4/1 -> mult4/2  "coeff_const4"
  adder_tree/2(dout) -> outport/1
  mult4/1 -> adder_tree/5(din_4)  "mult_out4"
  mult3/1 -> adder_tree/4(din_3)  "mult_out3"
  mult2/1 -> adder_tree/3(din_2)  "mult_out2"
  mult1/1 -> adder_tree/2(din_1)  "mult_out1"
  coeff_const5/1 -> adder_tree/1(sync)

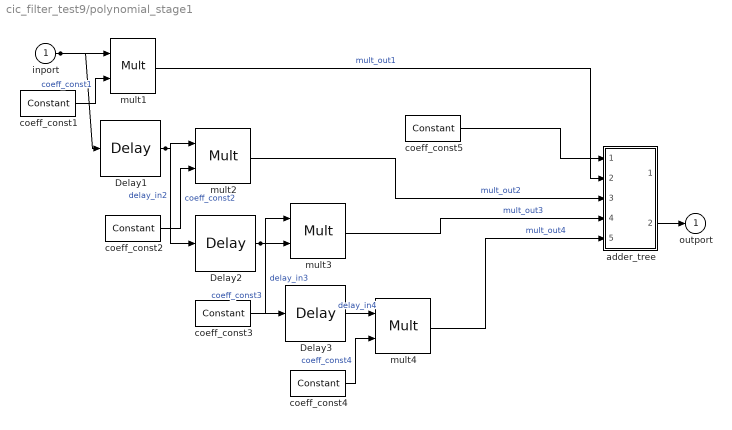
== system cic_filter_test9/polynomial_stage1 ==
  inport : Inport
  Delay1 : xbsIndex_r4/Delay  en=off  latency=1  dbl_ovrd=off  reg_retiming=off  block_type=delay
      settings: block_version=11.4
  Delay2 : xbsIndex_r4/Delay  en=off  latency=1  dbl_ovrd=off  reg_retiming=off  block_type=delay
      settings: block_version=11.4
  Delay3 : xbsIndex_r4/Delay  en=off  latency=1  dbl_ovrd=off  reg_retiming=off  block_type=delay
      settings: block_version=11.4
  adder_tree : Subsystem
  coeff_const1 : xbsIndex_r4/Constant  arith_type=Signed (2's comp)  const=1  n_bits=3  bin_pt=0  explicit_period=off  period=1  equ=P=C  opselect=C  inp2=PCIN>>17  opr=+  inp1=P  carry=CIN  dbl_ovrd=off  block_type=constant
      settings: block_version=11.4
  coeff_const2 : xbsIndex_r4/Constant  arith_type=Signed (2's comp)  const=3  n_bits=3  bin_pt=0  explicit_period=off  period=1  equ=P=C  opselect=C  inp2=PCIN>>17  opr=+  inp1=P  carry=CIN  dbl_ovrd=off  block_type=constant
      settings: block_version=11.4
  coeff_const3 : xbsIndex_r4/Constant  arith_type=Signed (2's comp)  const=3  n_bits=3  bin_pt=0  explicit_period=off  period=1  equ=P=C  opselect=C  inp2=PCIN>>17  opr=+  inp1=P  carry=CIN  dbl_ovrd=off  block_type=constant
      settings: block_version=11.4
  coeff_const4 : xbsIndex_r4/Constant  arith_type=Signed (2's comp)  const=1  n_bits=3  bin_pt=0  explicit_period=off  period=1  equ=P=C  opselect=C  inp2=PCIN>>17  opr=+  inp1=P  carry=CIN  dbl_ovrd=off  block_type=constant
      settings: block_version=11.4
  coeff_const5 : xbsIndex_r4/Constant  arith_type=Boolean  const=1  n_bits=6  bin_pt=0  explicit_period=on  period=1  equ=P=C  opselect=C  inp2=PCIN>>17  opr=+  inp1=P  carry=CIN  dbl_ovrd=off  block_type=constant
      settings: block_version=11.4
  mult{1..4} (4 alike) : xbsIndex_r4/Mult  precision=Full  arith_type="Signed  (2's comp)"  n_bits=9  bin_pt=0  quantization=Truncate  overflow=Wrap  en=off  latency=2  dbl_ovrd=off  use_behavioral_HDL=off  opt=Speed  use_embedded=on  optimum_pipeline=off  pipeline=on  use_rpm=on  placement_style=Triangular  block_type=mult
      settings: block_version=11.4
  outport : Outport
  wires:
  inport/1 -> Delay1/1, mult1/1
  Delay1/1 -> mult2/1, Delay2/1  "delay_in2"
  Delay2/1 -> Delay3/1, mult3/1  "delay_in3"
  Delay3/1 -> mult4/1  "delay_in4"
  coeff_const3/1 -> mult3/2  "coeff_const3"
  coeff_const1/1 -> mult1/2  "coeff_const1"
  coeff_const2/1 -> mult2/2  "coeff_const2"
  coeff_const4/1 -> mult4/2  "coeff_const4"
  adder_tree/2(dout) -> outport/1
  mult4/1 -> adder_tree/5(din_4)  "mult_out4"
  mult3/1 -> adder_tree/4(din_3)  "mult_out3"
  mult2/1 -> adder_tree/3(din_2)  "mult_out2"
  mult1/1 -> adder_tree/2(din_1)  "mult_out1"
  coeff_const5/1 -> adder_tree/1(sync)

== system cic_filter_test9/CIC Filter/Differentiator1 ==
  In1 : Inport  OutDataType=sfix(16)  OutScaling=2^0
  AddSub : xbsIndex_r4/AddSub  mode=Subtraction  use_carryin=off  use_carryout=off  en=off  latency=1  precision=User Defined  arith_type="Signed  (2's comp)"  n_bits=output_bitwidth  bin_pt=output_binpt  quantization=Truncate  overflow=Wrap  dbl_ovrd=off  use_behavioral_HDL=on  hw_selection=Fabric  pipelined=off  use_rpm=on  block_type=addsub
      settings: xl_area=[53 106 0 106 0 0 0]  block_version=VER_STRING_GOES_HERE
  Delay : xbsIndex_r4/Delay  en=off  latency=m  dbl_ovrd=off  reg_retiming=off  block_type=delay
      settings: infoedit="Delay line having  configurable length.<P><P>Hardware notes: A delay line is a chain, each link of which is an SRL16 followed by a flip-flop. If register retiming is enabled, the delay line is a chain of flip-flops."  xl_area=[53 106 0 0 0 0 0]  block_version=VER_STRING_GOES_HERE
  Out1 : Outport  OutDataType=sfix(16)  OutScaling=2^0
  wires:
  In1/1 -> Delay/1, AddSub/1
  AddSub/1 -> Out1/1
  Delay/1 -> AddSub/2

== system cic_filter_test9/CIC Filter/Differentiator2 ==
  In1 : Inport  OutDataType=sfix(16)  OutScaling=2^0
  AddSub : xbsIndex_r4/AddSub  mode=Subtraction  use_carryin=off  use_carryout=off  en=off  latency=1  precision=User Defined  arith_type="Signed  (2's comp)"  n_bits=output_bitwidth  bin_pt=output_binpt  quantization=Truncate  overflow=Wrap  dbl_ovrd=off  use_behavioral_HDL=on  hw_selection=Fabric  pipelined=off  use_rpm=on  block_type=addsub
      settings: xl_area=[53 106 0 106 0 0 0]  block_version=VER_STRING_GOES_HERE
  Delay : xbsIndex_r4/Delay  en=off  latency=m  dbl_ovrd=off  reg_retiming=off  block_type=delay
      settings: infoedit="Delay line having  configurable length.<P><P>Hardware notes: A delay line is a chain, each link of which is an SRL16 followed by a flip-flop. If register retiming is enabled, the delay line is a chain of flip-flops."  xl_area=[53 106 0 0 0 0 0]  block_version=VER_STRING_GOES_HERE
  Out1 : Outport  OutDataType=sfix(16)  OutScaling=2^0
  wires:
  Delay/1 -> AddSub/2
  AddSub/1 -> Out1/1
  In1/1 -> AddSub/1, Delay/1
